simulink model "task1_lab8"  (R2018a)
settings: Solver=VariableStepAuto  StartTime=0.0  StopTime=8  RelTol=1e-3
settings Model: Creator=muhsi  LastModifiedBy=muhsi

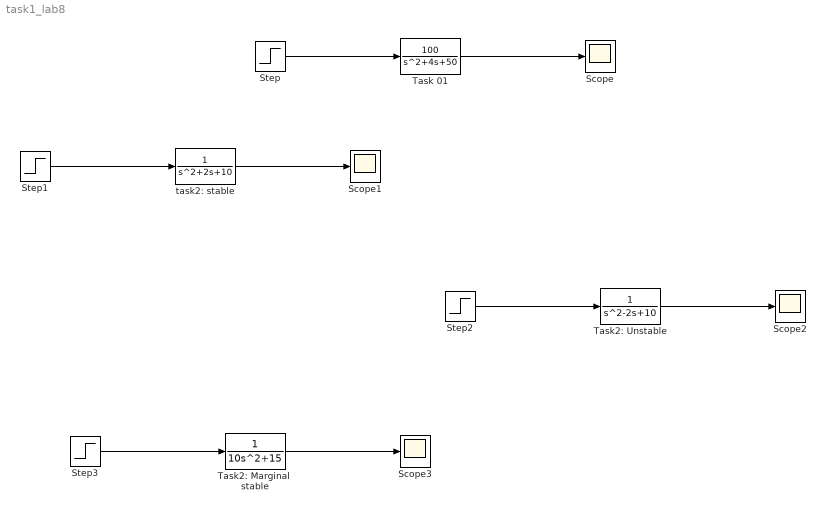
== system task1_lab8 ==
  Scope{,1..3} (4 alike) : Scope
  Step{,1..3} (4 alike) : Step  SampleTime=0
  "Task 01 " : TransferFcn  Numerator=[100]  Denominator=[1 4 50]
  "Task2: Marginal  stable " : TransferFcn  Denominator=[10 0 15]
  Task2: Unstable : TransferFcn  Denominator=[1 -2 10]
  "task2: stable " : TransferFcn  Denominator=[1 2 10]
  wires:
  Step/1 -> "Task 01 "/1
  "Task 01 "/1 -> Scope/1
  "task2: stable "/1 -> Scope1/1
  Step1/1 -> "task2: stable "/1
  Step2/1 -> Task2: Unstable/1
  Task2: Unstable/1 -> Scope2/1
  Step3/1 -> "Task2: Marginal  stable "/1
  "Task2: Marginal  stable "/1 -> Scope3/1
